simulink model "Quadcopter_Stabilize_LQI_Sim"  (R2016b)
settings: Solver=ode45  StartTime=0.0  StopTime=50  RelTol=1e-3  EnableMultiTasking=on
undefined symbols (not defined in the file or in its folder): A, B, C, DiscIntNeverNeededParam, g, K_lqi, m, Ts, X0
settings Model: Creator=Toshiba  LastModifiedBy=AAstudillo
settings DataIOCC: LimitDataPoints=on  SaveFormat=Array  SignalLoggingSaveFormat=ModelDataLogs
settings OptimizationCC: LifeSpan=inf
settings DebuggingCC: SolverPrmCheckMsg=warning  MultiTaskDSMMsg=warning  MultiTaskCondExecSysMsg=none  SFUnexpectedBacktrackingDiag=warning  SFNoUnconditionalDefaultTransitionDiag=warning  SFExecutionAtInitializationDiag=none
settings HardwareCC: ProdBitPerPointer=32  ProdBitPerSizeT=32  ProdBitPerPtrDiffT=32  ProdLargestAtomicFloat=None  ProdIntDivRoundTo=Undefined  ProdEndianess=Unspecified  ProdWordSize=32  ProdHWDeviceType=32-bit Generic
settings ModelReferenceCC: PropagateSignalLabelsOutOfModel=off
settings GRTTargetCC: TargetLangStandard=C89/C90 (ANSI)  GeneratePreprocessorConditionals=Disable all
settings ConfigComp: CovMetricSettings=dw  CovHtmlReporting=on  CovSaveCumulativeToWorkspaceVar=on  CovSaveSingleToWorkspaceVar=on  CovExternalEMLEnable=off

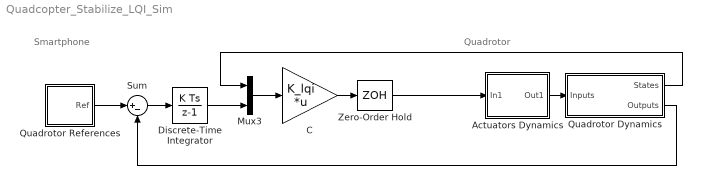
== system Quadcopter_Stabilize_LQI_Sim ==
  note: Quadrotor
  note: Smartphone
  Actuators Dynamics : Subsystem
  C : Gain  Gain=K_lqi  Multiplication=Matrix(K*u)
  Discrete-Time Integrator : DiscreteIntegrator  InitialConditionSetting=State (most efficient)  SampleTime=Ts  ICPrevOutput=DiscIntNeverNeededParam  ICPrevScaledInput=DiscIntNeverNeededParam
  Mux3 : Mux  Inputs=2
  Quadrotor Dynamics : Subsystem
  Quadrotor References : Subsystem
  Sum : Sum  Inputs=|+-
  Zero-Order Hold : ZeroOrderHold  SampleTime=Ts
  wires:
  C/1 -> Zero-Order Hold/1
  Quadrotor Dynamics/1(States) -> Mux3/1
  Mux3/1 -> C/1
  Quadrotor References/1(Ref) -> Sum/1
  Sum/1 -> Discrete-Time Integrator/1
  Discrete-Time Integrator/1 -> Mux3/2
  Quadrotor Dynamics/2(Outputs) -> Sum/2
  Zero-Order Hold/1 -> Actuators Dynamics/1(In1)
  Actuators Dynamics/1(Out1) -> Quadrotor Dynamics/1(Inputs)

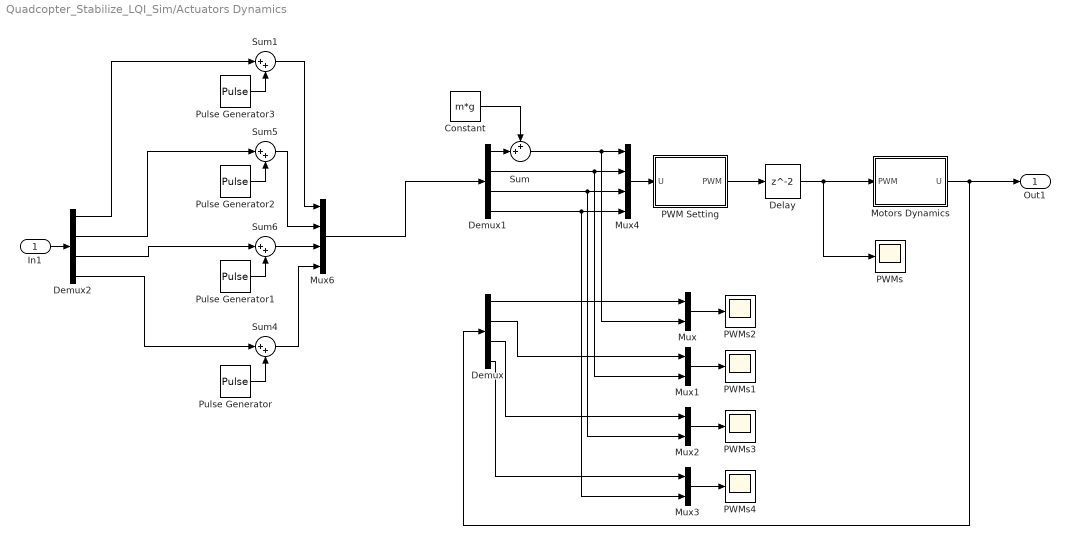
== system Quadcopter_Stabilize_LQI_Sim/Actuators Dynamics ==
  In1 : Inport
  Constant : Constant  Value=m*g  VectorParams1D=off
  Delay : Delay  SampleTime=Ts/10
  Demux : Demux
  Demux1 : Demux
  Demux2 : Demux
  Motors Dynamics : MATLAB Function  TreatAsAtomicUnit=on
  Mux{,1..3} (4 alike) : Mux  Inputs=2
  Mux4 : Mux
  Mux6 : Mux
  PWM Setting : MATLAB Function  TreatAsAtomicUnit=on
  PWMs{,1..4} (5 alike) : Scope
  Pulse Generator : DiscretePulseGenerator  PulseType=Time based  Amplitude=0.2  Period=20  PulseWidth=10  PhaseDelay=10
  Pulse Generator1 : DiscretePulseGenerator  PulseType=Time based  Amplitude=0.2  Period=15  PulseWidth=10  PhaseDelay=5
  Pulse Generator2 : DiscretePulseGenerator  PulseType=Time based  Amplitude=0.5  Period=17  PhaseDelay=15
  Pulse Generator3 : DiscretePulseGenerator  PulseType=Time based  Period=15  PhaseDelay=15
  Sum : Sum  Inputs=++|
  Sum{1,4..6} (4 alike) : Sum  Inputs=|++
  Out1 : Outport
  wires:
  Motors Dynamics/1(U) -> Demux/1, Out1/1
  Mux/1 -> PWMs2/1
  Mux1/1 -> PWMs1/1
  Mux2/1 -> PWMs3/1
  Mux3/1 -> PWMs4/1
  Demux/1 -> Mux/1
  Demux/2 -> Mux1/1
  Demux/3 -> Mux2/1
  Demux/4 -> Mux3/1
  Constant/1 -> Sum/1
  Demux1/1 -> Sum/2
  Sum/1 -> Mux/2, Mux4/1
  Demux1/2 -> Mux1/2, Mux4/2
  Demux1/3 -> Mux2/2, Mux4/3
  Demux1/4 -> Mux3/2, Mux4/4
  Mux4/1 -> PWM Setting/1(U)
  PWM Setting/1(PWM) -> Delay/1
  Delay/1 -> PWMs/1, Motors Dynamics/1(PWM)
  Pulse Generator/1 -> Sum4/2
  Pulse Generator1/1 -> Sum6/2
  Pulse Generator2/1 -> Sum5/2
  In1/1 -> Demux2/1
  Demux2/2 -> Sum5/1
  Demux2/3 -> Sum6/1
  Demux2/4 -> Sum4/1
  Sum5/1 -> Mux6/2
  Sum6/1 -> Mux6/3
  Sum4/1 -> Mux6/4
  Pulse Generator3/1 -> Sum1/2
  Demux2/1 -> Sum1/1
  Sum1/1 -> Mux6/1
  Mux6/1 -> Demux1/1

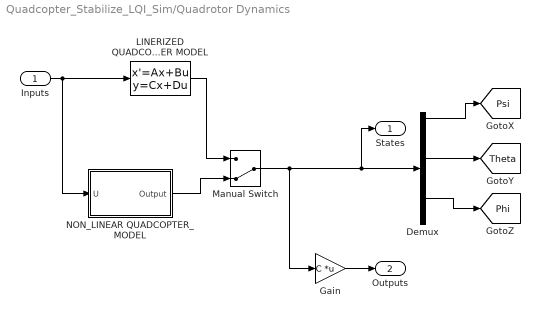
== system Quadcopter_Stabilize_LQI_Sim/Quadrotor Dynamics ==
  Inputs : Inport
  Demux : Demux  Outputs=6
  Gain : Gain  Gain=C  Multiplication=Matrix(K*u)
  LINERIZED QUADCOPTER MODEL : StateSpace  A=A  B=B  C=eye(6)  D=zeros(6,4)  X0=X0
  Manual Switch : ManualSwitch  CurrentSetting=0
  NON_LINEAR QUADCOPTER_MODEL : Subsystem
  States : Outport
  Outputs : Outport  Port=2
  tag scope: Phi=global, Psi=global, Theta=global
  wires:
  Inputs/1 -> LINERIZED QUADCOPTER MODEL/1, NON_LINEAR QUADCOPTER_MODEL/1(U)
  LINERIZED QUADCOPTER MODEL/1 -> Manual Switch/1
  Manual Switch/1 -> Gain/1, States/1, Demux/1
  NON_LINEAR QUADCOPTER_MODEL/1("Output ") -> Manual Switch/2
  Demux/1 -> [Psi]
  Demux/5 -> [Phi]
  Demux/3 -> [Theta]
  Gain/1 -> Outputs/1

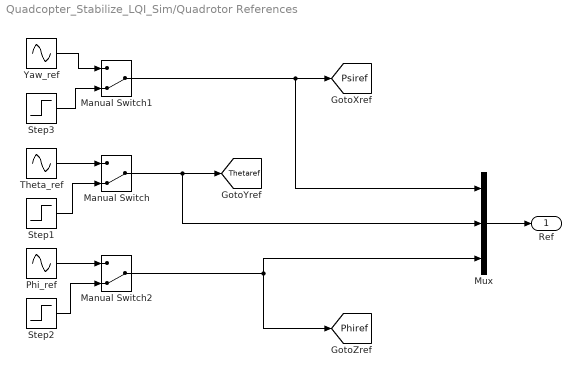
== system Quadcopter_Stabilize_LQI_Sim/Quadrotor References ==
  Manual Switch : ManualSwitch  CurrentSetting=0
  Manual Switch1 : ManualSwitch  CurrentSetting=0
  Manual Switch2 : ManualSwitch  CurrentSetting=0
  Mux : Mux  Inputs=3
  Phi_ref : Sin  Amplitude=10*pi/180  Frequency=3.141592654*0.05  Phase=3.141592654  SampleTime=Ts
  Step1 : Step  Time=15  After=10*pi/180  SampleTime=Ts
  Step2 : Step  Time=20  After=-10*pi/180  SampleTime=Ts
  Step3 : Step  Time=25  After=10*pi/180  SampleTime=Ts
  Theta_ref : Sin  Amplitude=10*pi/180  Frequency=3.141592654*0.1  Phase=3.141592654/2  SampleTime=Ts
  Yaw_ref : Sin  Amplitude=10*pi/180  Frequency=3.141592654*0.1  SampleTime=Ts
  Ref : Outport
  tag scope: Phiref=global, Psiref=global, Thetaref=global
  wires:
  Mux/1 -> Ref/1
  Yaw_ref/1 -> Manual Switch1/1
  Manual Switch1/1 -> [Psiref], Mux/1
  Step3/1 -> Manual Switch1/2
  Theta_ref/1 -> Manual Switch/1
  Step1/1 -> Manual Switch/2
  Manual Switch/1 -> Mux/2, [Thetaref]
  Step2/1 -> Manual Switch2/2
  Phi_ref/1 -> Manual Switch2/1
  Manual Switch2/1 -> Mux/3, [Phiref]

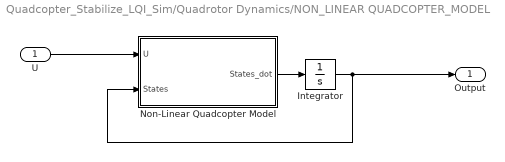
== system Quadcopter_Stabilize_LQI_Sim/Quadrotor Dynamics/NON_LINEAR QUADCOPTER_MODEL ==
  U : Inport
  Integrator : Integrator  InitialCondition=X0
  Non-Linear Quadcopter Model : MATLAB Function  TreatAsAtomicUnit=on
  "Output " : Outport
  wires:
  Non-Linear Quadcopter Model/1(States_dot) -> Integrator/1
  U/1 -> Non-Linear Quadcopter Model/1(U)
  Integrator/1 -> "Output "/1, Non-Linear Quadcopter Model/2(States)

== matlab function Quadcopter_Stabilize_LQI_Sim/Actuators Dynamics/PWM Setting ==
  data: U input; PWM output
function PWM = fcn(U)

M_inv = [0.2500  11.9048   -1.4490   -1.4490;
        0.2500  -11.9048   -1.4490    1.4490;
        0.2500   11.9048    1.4490    1.4490;
        0.2500  -11.9048    1.4490   -1.4490];

Force = M_inv*U;

% if Force(1) < 0
%     Force(3) = Force(3) - Force(1);
% end
% if Force(2) < 0
%     Force(4) = Force(4) - Force(2);
% end
% if Force(3) < 0
%     Force(1) = Force(1) - Force(3);
% end
% if Force(4) < 0
%     Force(2) = Force(2) - Force(4);
% end

PWM_1 =  -1.983*(Force(1)^2) + 47.84*Force(1) + 3.835; % PWM [0...255]
PWM_2 =  -1.983*(Force(2)^2) + 47.84*Force(2) + 3.835; % PWM [0...255]
PWM_3 =  -1.983*(Force(3)^2) + 47.84*Force(3) + 3.835; % PWM [0...255]
PWM_4 =  -1.983*(Force(4)^2) + 47.84*Force(4) + 3.835; % PWM [0...255]

if PWM_1 < 0
    PWM_3 = PWM_3 - PWM_1;
end
if PWM_2 < 0
    PWM_4 = PWM_4  - PWM_2;
end
if PWM_3 < 0
    PWM_1 = PWM_1 - PWM_3;
end
if Force(4) < 0
    PWM_2 = PWM_2 - PWM_4 ;
end

PWM_1 = min(255, max(0, PWM_1));
PWM_2 = min(255, max(0, PWM_2));
PWM_3 = min(255, max(0, PWM_3));
PWM_4 = min(255, max(0, PWM_4));

PWM = [PWM_1 PWM_2 PWM_3 PWM_4];

== matlab function Quadcopter_Stabilize_LQI_Sim/Quadrotor Dynamics/NON_LINEAR QUADCOPTER_MODEL/Non-Linear Quadcopter Model ==
  data: U input; States input; States_dot output
function States_dot  = fcn(U, States)

% Gravity constant
              g = 9.807;

              m = 1.568;
              Ixx = 0.0135;
              Iyy = 0.0124;
              Izz = 0.0336;

    %Inputs = U, States
    %Outputs = States_dot  
    %States: X dX Y dY Z dZ Psi dPsi Theta dTheta Phi dPhi
    %        1  2 3  4 5  6  7   8     9      10   11  12
    
    U1 = U(1);
    U2 = U(2);
    U3 = U(3);
    U4 = U(4);

    dPsi = States(2);
    ddPsi = (((Ixx-Iyy)/Izz)*States(6)*States(4)) + (U2/Izz);
    dTheta = States(4);
    ddTheta = (((Izz-Ixx)/Iyy)*States(6)*States(2)) + (U3/Iyy);
    dPhi = States(6);
    ddPhi = (((Iyy-Izz)/Ixx)*States(4)*States(2)) + (U4/Ixx);

    States_dot = [dPsi, ddPsi, dTheta, ddTheta, dPhi, ddPhi]';

== matlab function Quadcopter_Stabilize_LQI_Sim/Actuators Dynamics/Motors Dynamics ==
  data: PWM input; U output
function U = fcn(PWM)

F_M1 = (5.441e-5)*(PWM(1)^2) + 0.01586*PWM(1) + 0.014808;
F_M2 = (5.441e-5)*(PWM(2)^2) + 0.01586*PWM(2) + 0.014808;
F_M3 = (5.441e-5)*(PWM(3)^2) + 0.01586*PWM(3) + 0.014808;
F_M4 = (5.441e-5)*(PWM(4)^2) + 0.01586*PWM(4) + 0.014808;

Force = [F_M1 F_M2*1.0256 F_M3 F_M4*1.0256]'; % CCW motors have 2.56 % more efficiency than CW motors

M = [1.0000    1.0000    1.0000    1.0000;
    0.0210   -0.0210    0.0210   -0.0210;
   -0.1725   -0.1725    0.1725    0.1725;
   -0.1725    0.1725    0.1725   -0.1725];


U = M*Force;
